simulink model "TestBed"  (R2015a)
settings: configuration reference "SIMULATION_CONFIGURATION" (kept outside this file)
settings Model: Creator=moritz  LastModifiedBy=moritz
settings ConfigSetRef: SourceLocation=Base Workspace

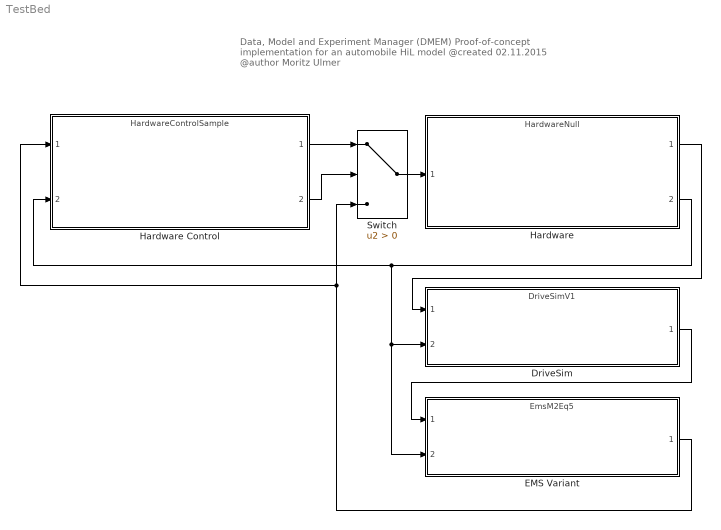
== system TestBed ==
  note: Data, Model and Experiment Manager (DMEM)
      | Proof-of-concept implementation for an automobile HiL model
      | @created 02.11.2015
      | @author Moritz Ulmer
  DriveSim : ModelReference  ModelNameDialog=DriveSimV1.slx  Variant=on  ModelReferenceVersion=1.48  CopyOfModelName=DriveSimV1.slx  DefaultDataLogging=on
  EMS Variant : ModelReference  ModelNameDialog=EmsM2Eq5.mdl  Variant=on  ModelReferenceVersion=1.26  CopyOfModelName=EmsM2Eq5.mdl  DefaultDataLogging=on
      settings: AttributesFormatString=%<ActiveVariant>
  Hardware : ModelReference  ModelNameDialog=HardwareNull  Variant=on  ModelReferenceVersion=1.2  CopyOfModelName=HardwareNull  DefaultDataLogging=on
  Hardware Control : ModelReference  DialogController=Simulink.DDGSource  ModelNameDialog=HardwareControlSample  Variant=on  ModelReferenceVersion=1.23  CopyOfModelName=HardwareControlSample
      settings: AttributesFormatString=%<ActiveVariant>
  Switch : Switch  Criteria=u2 > Threshold
  wires:
  DriveSim/1 -> EMS Variant/1
  EMS Variant/1 -> Switch/3, Hardware Control/1
  Hardware/2 -> Hardware Control/2, EMS Variant/2, DriveSim/2
  Hardware/1 -> DriveSim/1
  Switch/1 -> Hardware/1
  Hardware Control/2 -> Switch/2
  Hardware Control/1 -> Switch/1
